simulink library "BEML_EMU_CBTCInterface_Lib"  (R2019b)
settings: Solver=VariableStepAuto  StartTime=0.0  StopTime=10.0  RelTol=1e-3
undefined symbols (not defined in the file): ATCCabActivation, ATCSBResetIndication, ATCZeroSpeed, ATOBrake, ATONotBrake, ATOStartIndication, ATOState, ATOTBDemand, ATOTraction, CabActive, DMI, Door1Inhibited, Door2Inhibited, Door3Inhibited, Door4Inhibited, Electrical, EmergencyDetrainmentDoorLocked, LeftDoorCloseATCReq, LeftDoorCloseIndicator, LeftDoorOpenATCReq, LeftHoldDoorClose, LeftSideDoorCloseRequest, LeftSideDoorEnable, LeftSideDoorOpenRequest, NeutralSection, NoEmergencyBrakeOrder, NoServiceBrake, NotImmobilise, OnBoard, Platform, PowerOn, RightDoorCloseATCReq, RightDoorCloseIndicator, RightDoorOpenATCReq, RightHoldDoorClose, RightSideDoorCloseRequest, RightSideDoorEnable, RightSideDoorOpenRequest, RollbackDetected, ROSIndication, TCMS, TractionForward, u2, u3, u4, UTOModeActive, UTOPBIndicator, WakeUpCommand
libraries: simulink x8, LatchesLib x4
settings Model: Creator=rleighton  LastModifiedBy=hinganes
settings DataIOCC: ReturnWorkspaceOutputs=off
settings DebuggingCC: ArithmeticOperatorsInVariantConditions=warning
settings SFSimCC: SimUseLocalCustomCode=off  CustomCodeUndefinedFunction=UseInterfaceOnly
settings RTWCC: RTWUseLocalCustomCode=off

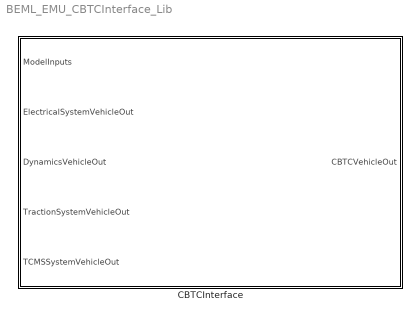
== system BEML_EMU_CBTCInterface_Lib ==
  CBTCInterface : Subsystem  SystemSampleTime=0.001

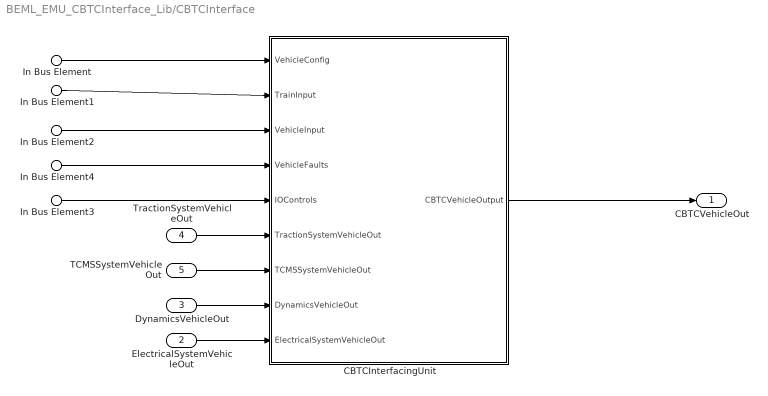
== system BEML_EMU_CBTCInterface_Lib/CBTCInterface ==
  In Bus Element : Inport  PortName=ModelInputs  Element=ProcessedVehicleConfig
  In Bus Element1 : Inport  PortName=ModelInputs  Element=ProcessedTrainInput
  In Bus Element2 : Inport  PortName=ModelInputs  Element=ProcessedVehicleInput
  In Bus Element4 : Inport  PortName=ModelInputs  Element=VehicleModelFaults
  In Bus Element3 : Inport  PortName=ModelInputs  Element=InputControlStates
  ElectricalSystemVehicleOut : Inport  Port=2
  DynamicsVehicleOut : Inport  Port=3
  TractionSystemVehicleOut : Inport  Port=4
  TCMSSystemVehicleOut : Inport  Port=5
  CBTCInterfacingUnit : Subsystem  TreatAsAtomicUnit=on  SystemSampleTime=0.01
  CBTCVehicleOut : Outport  VectorParamsAs1DForOutWhenUnconnected=off
  wires:
  In Bus Element3/1 -> CBTCInterfacingUnit/5(IOControls)
  CBTCInterfacingUnit/1(CBTCVehicleOutput) -> CBTCVehicleOut/1
  TractionSystemVehicleOut/1 -> CBTCInterfacingUnit/6(TractionSystemVehicleOut)
  TCMSSystemVehicleOut/1 -> CBTCInterfacingUnit/7(TCMSSystemVehicleOut)
  In Bus Element/1 -> CBTCInterfacingUnit/1(VehicleConfig)
  In Bus Element4/1 -> CBTCInterfacingUnit/4(VehicleFaults)
  In Bus Element2/1 -> CBTCInterfacingUnit/3(VehicleInput)
  In Bus Element1/1 -> CBTCInterfacingUnit/2(TrainInput)
  DynamicsVehicleOut/1 -> CBTCInterfacingUnit/8(DynamicsVehicleOut)
  ElectricalSystemVehicleOut/1 -> CBTCInterfacingUnit/9(ElectricalSystemVehicleOut)

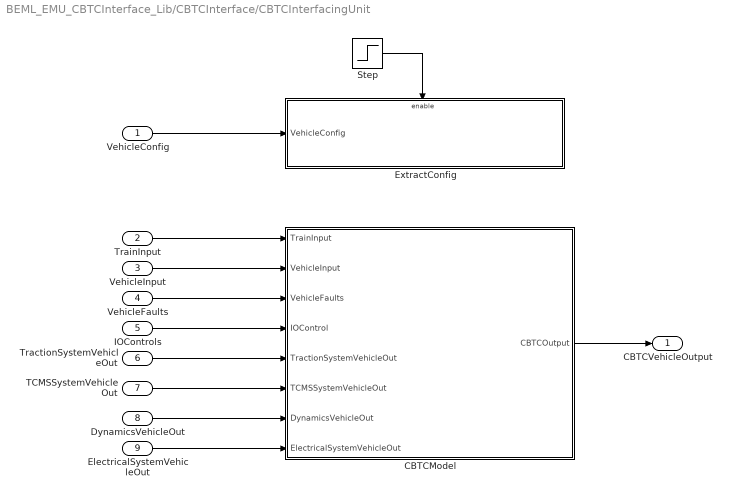
== system BEML_EMU_CBTCInterface_Lib/CBTCInterface/CBTCInterfacingUnit ==
  VehicleConfig : Inport  SampleTime=0.01
  TrainInput : Inport  Port=2  SampleTime=0.01
  VehicleInput : Inport  Port=3  SampleTime=0.01
  VehicleFaults : Inport  Port=4  SampleTime=0.01
  IOControls : Inport  Port=5
  TractionSystemVehicleOut : Inport  Port=6  SampleTime=0.01
  TCMSSystemVehicleOut : Inport  Port=7  SampleTime=0.01
  DynamicsVehicleOut : Inport  Port=8  SampleTime=0.01
  ElectricalSystemVehicleOut : Inport  Port=9  SampleTime=0.01
  CBTCModel : Subsystem
  ExtractConfig : Subsystem
  Step : Step  Before=1  After=0
  CBTCVehicleOutput : Outport  VectorParamsAs1DForOutWhenUnconnected=off
  wires:
  IOControls/1 -> CBTCModel/4(IOControl)
  TrainInput/1 -> CBTCModel/1(TrainInput)
  VehicleInput/1 -> CBTCModel/2(VehicleInput)
  TractionSystemVehicleOut/1 -> CBTCModel/5(TractionSystemVehicleOut)
  TCMSSystemVehicleOut/1 -> CBTCModel/6(TCMSSystemVehicleOut)
  VehicleConfig/1 -> ExtractConfig/1(VehicleConfig)
  Step/1 -> ExtractConfig/Enable
  VehicleFaults/1 -> CBTCModel/3(VehicleFaults)
  CBTCModel/1(CBTCOutput) -> CBTCVehicleOutput/1
  DynamicsVehicleOut/1 -> CBTCModel/7(DynamicsVehicleOut)
  ElectricalSystemVehicleOut/1 -> CBTCModel/8(ElectricalSystemVehicleOut)

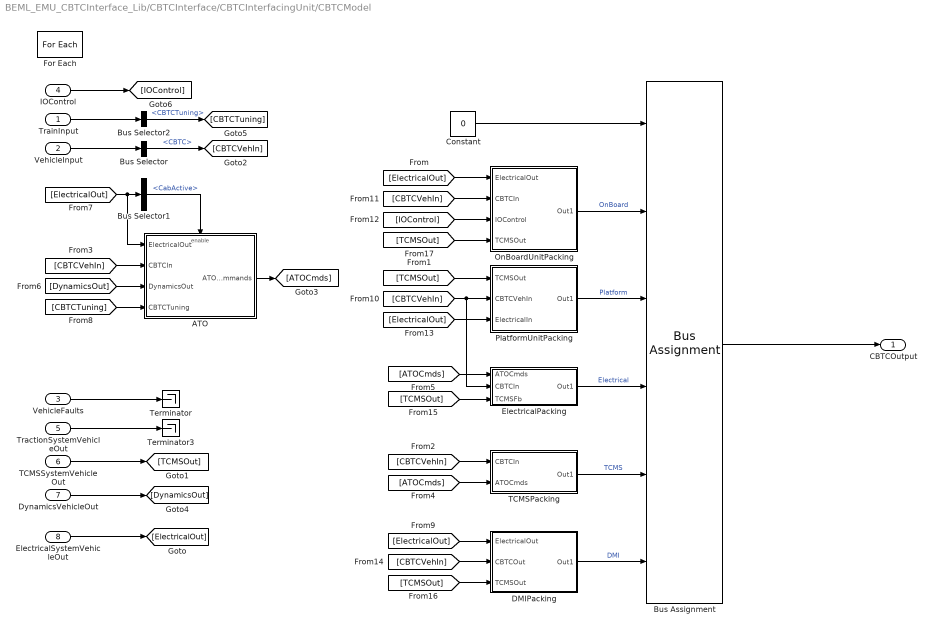
== system BEML_EMU_CBTCInterface_Lib/CBTCInterface/CBTCInterfacingUnit/CBTCModel ==
  TrainInput : Inport
  VehicleInput : Inport  Port=2  Partition=on  PartitionDimension=1  PartitionWidth=1  PartitionOffset=0
  VehicleFaults : Inport  Port=3  Partition=on  PartitionDimension=1  PartitionWidth=1  PartitionOffset=0
  IOControl : Inport  Port=4  Partition=on  PartitionDimension=1  PartitionWidth=1  PartitionOffset=0
  TractionSystemVehicleOut : Inport  Port=5  Partition=on  PartitionDimension=1  PartitionWidth=1  PartitionOffset=0
  TCMSSystemVehicleOut : Inport  Port=6  Partition=on  PartitionDimension=1  PartitionWidth=1  PartitionOffset=0
  DynamicsVehicleOut : Inport  Port=7  Partition=on  PartitionDimension=1  PartitionWidth=1  PartitionOffset=0
  ElectricalSystemVehicleOut : Inport  Port=8  Partition=on  PartitionDimension=1  PartitionWidth=1  PartitionOffset=0
  ATO : Subsystem
  Bus Assignment : BusAssignment  AssignedSignals=OnBoard,Platform,Electrical,TCMS,DMI
  Bus Selector : BusSelector  OutputSignals=CBTC
  Bus Selector1 : BusSelector  OutputSignals=TCMS.CabActive
  Bus Selector2 : BusSelector  OutputSignals=CBTCTuning
  Constant : Constant  Value=0  OutDataTypeStr=Bus: BD_CBTC_Out_Vehicle
  DMIPacking : Subsystem
  ElectricalPacking : Subsystem
  For Each : ForEach  DisableCoverage=on
  OnBoardUnitPacking : Subsystem
  PlatformUnitPacking : Subsystem
  TCMSPacking : Subsystem
  Terminator : Terminator
  Terminator3 : Terminator
  CBTCOutput : Outport  ConcatenationDimension=1  VectorParamsAs1DForOutWhenUnconnected=off
  wires:
  [TCMSOut] -> OnBoardUnitPacking/4(TCMSOut)
  [TCMSOut] -> DMIPacking/3(TCMSOut)
  [TCMSOut] -> ElectricalPacking/3(TCMSFb)
  [CBTCVehIn] -> DMIPacking/2(CBTCOut)
  [ElectricalOut] -> PlatformUnitPacking/3(ElectricalIn)
  [IOControl] -> OnBoardUnitPacking/3(IOControl)
  IOControl/1 -> [IOControl]
  [CBTCVehIn] -> OnBoardUnitPacking/2(CBTCIn)
  [CBTCVehIn] -> PlatformUnitPacking/2(CBTCVehIn), ElectricalPacking/2(CBTCIn)
  ElectricalSystemVehicleOut/1 -> [ElectricalOut]
  Bus Assignment/1 -> CBTCOutput/1
  Bus Selector/1 -> [CBTCVehIn]  "<CBTC>"
  TrainInput/1 -> Bus Selector2/1
  VehicleInput/1 -> Bus Selector/1
  VehicleFaults/1 -> Terminator/1
  TractionSystemVehicleOut/1 -> Terminator3/1
  TCMSSystemVehicleOut/1 -> [TCMSOut]
  DynamicsVehicleOut/1 -> [DynamicsOut]
  OnBoardUnitPacking/1(Out1) -> Bus Assignment/2  "OnBoard"
  [ElectricalOut] -> OnBoardUnitPacking/1(ElectricalOut)
  Constant/1 -> Bus Assignment/1
  PlatformUnitPacking/1(Out1) -> Bus Assignment/3  "Platform"
  [TCMSOut] -> PlatformUnitPacking/1(TCMSOut)
  ElectricalPacking/1(Out1) -> Bus Assignment/4  "Electrical"
  TCMSPacking/1(Out1) -> Bus Assignment/5  "TCMS"
  [CBTCVehIn] -> TCMSPacking/1(CBTCIn)
  [CBTCVehIn] -> ATO/2(CBTCIn)
  ATO/1(ATOCommands) -> [ATOCmds]
  [ATOCmds] -> TCMSPacking/2(ATOCmds)
  [ATOCmds] -> ElectricalPacking/1(ATOCmds)
  [DynamicsOut] -> ATO/3(DynamicsOut)
  [ElectricalOut] -> ATO/1(ElectricalOut), Bus Selector1/1
  Bus Selector1/1 -> ATO/Enable  "<CabActive>"
  Bus Selector2/1 -> [CBTCTuning]  "<CBTCTuning>"
  [CBTCTuning] -> ATO/4(CBTCTuning)
  DMIPacking/1(Out1) -> Bus Assignment/6  "DMI"
  [ElectricalOut] -> DMIPacking/1(ElectricalOut)

== system BEML_EMU_CBTCInterface_Lib/CBTCInterface/CBTCInterfacingUnit/ExtractConfig ==
  VehicleConfig : Inport
  Enable : EnablePort
  ExtractConfig : Subsystem
  wires:
  VehicleConfig/1 -> ExtractConfig/1(VehicleConfig)

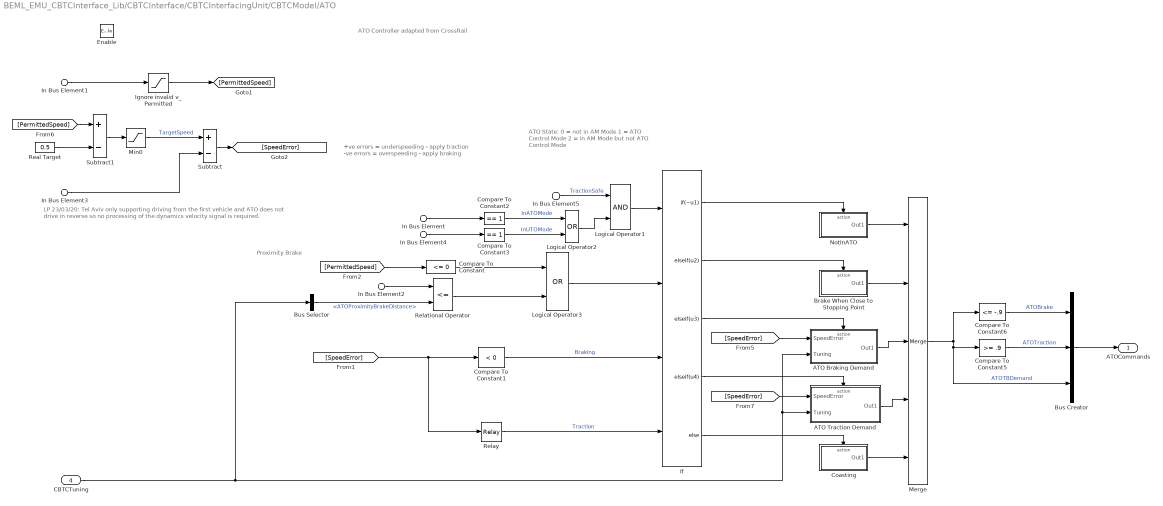
== system BEML_EMU_CBTCInterface_Lib/CBTCInterface/CBTCInterfacingUnit/CBTCModel/ATO ==
  note: ATO Controller adapted from CrossRail
  note: ATO State:
      | 0 = not in AM Mode
      | 1 = ATO Control Mode
      | 2 = in AM Mode but not ATO Control Mode
  note: +ve errors = underspeeding - apply traction
      | -ve errors = overspeeding - apply braking
  note: LP 23/03/20: Tel Aviv only supporting driving from the first vehicle and ATO does
      | not drive in reverse so no processing of the dynamics velocity signal is required.
  note: Proximity Brake
  In Bus Element5 : Inport  PortName=ElectricalOut  Element=Traction.TractionSafe
  In Bus Element : Inport  Port=2  PortName=CBTCIn  Element=OnBoard.ATOState
  In Bus Element1 : Inport  Port=2  PortName=CBTCIn  Element=OnBoard.ATOPermittedSpeed
  In Bus Element2 : Inport  Port=2  PortName=CBTCIn  Element=OnBoard.ATOPermittedDistance
  In Bus Element4 : Inport  Port=2  PortName=CBTCIn  Element=OnBoard.UTOModeActive
  In Bus Element3 : Inport  Port=3  PortName=DynamicsOut  Element=Inertia.Velocity
  CBTCTuning : Inport  Port=4
  Enable : EnablePort  StatesWhenEnabling=reset
  ATO Braking Demand : Subsystem  TreatAsAtomicUnit=on
  ATO Traction Demand : Subsystem  TreatAsAtomicUnit=on
  Brake When Close to Stopping Point : Subsystem  TreatAsAtomicUnit=on
  Bus Creator : BusCreator  Inputs=3
  Bus Selector : BusSelector  OutputSignals=ATOProximityBrakeDistance
  Coasting : Subsystem  TreatAsAtomicUnit=on
  Compare To Constant : simulink/Logic and Bit Operations/Compare To Constant  relop=<=  const=0  OutDataTypeStr=boolean
  Compare To Constant1 : simulink/Logic and Bit Operations/Compare To Constant  relop=<  const=0  OutDataTypeStr=boolean
  Compare To Constant2 : simulink/Logic and Bit Operations/Compare To Constant  relop===  const=1  OutDataTypeStr=boolean
  Compare To Constant3 : simulink/Logic and Bit Operations/Compare To Constant  relop===  const=1  OutDataTypeStr=boolean
  Compare To Constant5 : simulink/Logic and Bit Operations/Compare To Constant  relop=>=  const=.9  OutDataTypeStr=boolean
  Compare To Constant6 : simulink/Logic and Bit Operations/Compare To Constant  relop=<=  const=-.9  OutDataTypeStr=boolean
  If : If  NumInputs=4  IfExpression=~u1  ElseIfExpressions=u2,u3,u4
  Ignore invalid v_Permitted : Saturate  UpperLimit=80/3.6  LowerLimit=0
  Logical Operator1 : Logic  AllPortsSameDT=off  OutDataTypeStr=boolean
  Logical Operator2 : Logic  Operator=OR  AllPortsSameDT=off  OutDataTypeStr=boolean
  Logical Operator3 : Logic  Operator=OR  AllPortsSameDT=off  OutDataTypeStr=boolean
  Merge : Merge  Inputs=5
  Min0 : Saturate  UpperLimit=inf  LowerLimit=0
  NotInATO : Subsystem  TreatAsAtomicUnit=on
  Real Target : Constant  Value=0.5
  Relational Operator : RelationalOperator  Operator=<=  OutDataTypeStr=boolean  RndMeth=Simplest
  Relay : Relay  OnSwitchValue=0.5  OffSwitchValue=0.05  OutDataTypeStr=boolean
  Subtract : Sum  Inputs=+-
  Subtract1 : Sum  Inputs=+-
  ATOCommands : Outport
  wires:
  In Bus Element4/1 -> Compare To Constant3/1
  Compare To Constant3/1 -> Logical Operator2/2  "InUTOMode"
  Logical Operator2/1 -> Logical Operator1/2
  Compare To Constant2/1 -> Logical Operator2/1  "InATOMode"
  Merge/1 -> Bus Creator/3, Compare To Constant5/1, Compare To Constant6/1  "ATOTBDemand"
  Bus Creator/1 -> ATOCommands/1
  Relational Operator/1 -> Logical Operator3/2
  ATO Braking Demand/1(Out1) -> Merge/3
  Compare To Constant5/1 -> Bus Creator/2  "ATOTraction"
  Compare To Constant6/1 -> Bus Creator/1  "ATOBrake"
  [SpeedError] -> Relay/1, Compare To Constant1/1
  CBTCTuning/1 -> ATO Braking Demand/2(Tuning), ATO Traction Demand/2(Tuning), Bus Selector/1
  Compare To Constant1/1 -> If/3  "Braking"
  If/3 -> ATO Braking Demand/Action
  Ignore invalid v_Permitted/1 -> [PermittedSpeed]
  Subtract/1 -> [SpeedError]
  Relay/1 -> If/4  "Traction"
  [SpeedError] -> ATO Braking Demand/1(SpeedError)
  In Bus Element2/1 -> Relational Operator/1
  Compare To Constant/1 -> Logical Operator3/1
  If/4 -> ATO Traction Demand/Action
  Logical Operator3/1 -> If/2
  [SpeedError] -> ATO Traction Demand/1(SpeedError)
  In Bus Element3/1 -> Subtract/2
  In Bus Element1/1 -> Ignore invalid v_Permitted/1
  If/5 -> Coasting/Action
  ATO Traction Demand/1(Out1) -> Merge/4
  If/2 -> Brake When Close to Stopping Point/Action
  Real Target/1 -> Subtract1/2
  Brake When Close to Stopping Point/1(Out1) -> Merge/2
  Coasting/1(Out1) -> Merge/5
  [PermittedSpeed] -> Compare To Constant/1
  [PermittedSpeed] -> Subtract1/1
  If/1 -> NotInATO/Action
  NotInATO/1(Out1) -> Merge/1
  Logical Operator1/1 -> If/1
  Min0/1 -> Subtract/1  "TargetSpeed"
  In Bus Element5/1 -> Logical Operator1/1  "TractionSafe"
  In Bus Element/1 -> Compare To Constant2/1
  Subtract1/1 -> Min0/1
  Bus Selector/1 -> Relational Operator/2  "<ATOProximityBrakeDistance>"

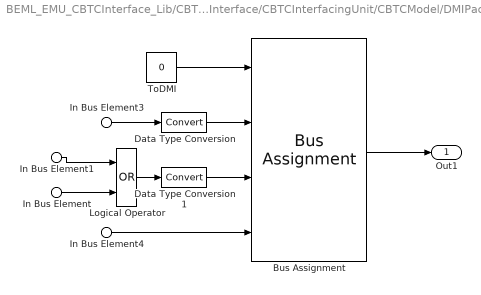
== system BEML_EMU_CBTCInterface_Lib/CBTCInterface/CBTCInterfacingUnit/CBTCModel/DMIPacking ==
  In Bus Element1 : Inport  PortName=ElectricalOut  Element=SignalSys.CabActive
  In Bus Element3 : Inport  PortName=ElectricalOut  Element=SignalSys.DMIPower
  In Bus Element : Inport  Port=2  PortName=CBTCOut  Element=OnBoard.ATCCabActivation
  In Bus Element4 : Inport  Port=3  PortName=TCMSOut  Element=Control.ElectricalSystem.TrainInNeutralSection
  Bus Assignment : BusAssignment  AssignedSignals=PowerOn,CabActive,NeutralSection
  Data Type Conversion : DataTypeConversion
  Data Type Conversion1 : DataTypeConversion
  Logical Operator : Logic  Operator=OR  AllPortsSameDT=off  OutDataTypeStr=boolean
  ToDMI : Constant  Value=0  OutDataTypeStr=Bus: BD_CBTC_Out_Vehicle_DMI
  Out1 : Outport
  wires:
  In Bus Element4/1 -> Bus Assignment/4
  In Bus Element/1 -> Logical Operator/2
  Logical Operator/1 -> Data Type Conversion1/1
  Data Type Conversion1/1 -> Bus Assignment/3
  Data Type Conversion/1 -> Bus Assignment/2
  Bus Assignment/1 -> Out1/1
  ToDMI/1 -> Bus Assignment/1
  In Bus Element1/1 -> Logical Operator/1
  In Bus Element3/1 -> Data Type Conversion/1

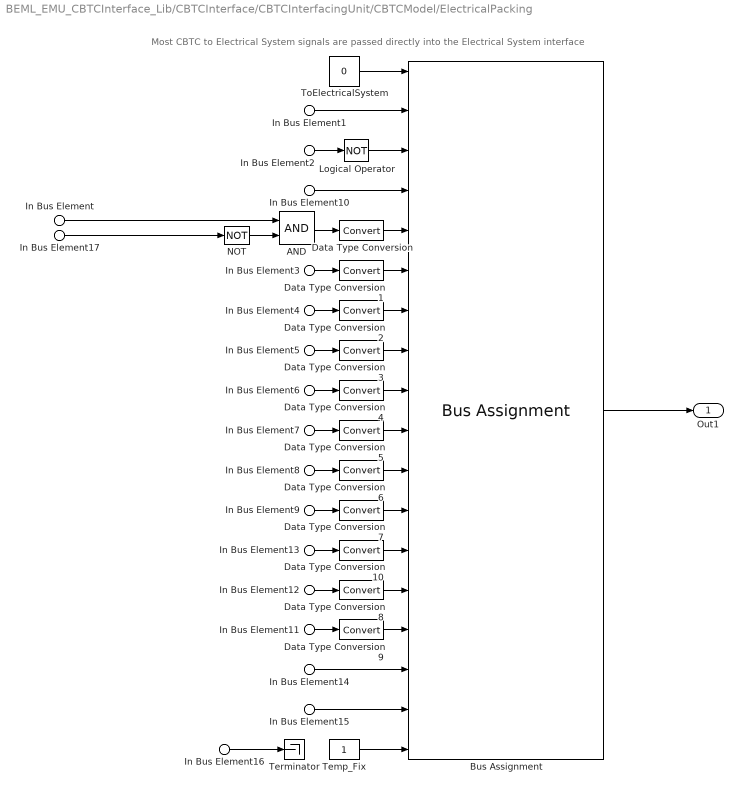
== system BEML_EMU_CBTCInterface_Lib/CBTCInterface/CBTCInterfacingUnit/CBTCModel/ElectricalPacking ==
  note: Most CBTC to Electrical System signals are passed directly into the Electrical System interface
  In Bus Element1 : Inport  PortName=ATOCmds  Element=ATOTraction
  In Bus Element2 : Inport  PortName=ATOCmds  Element=ATOBrake
  In Bus Element10 : Inport  PortName=ATOCmds  Element=ATOTBDemand
  In Bus Element : Inport  Port=2  PortName=CBTCIn  Element=OnBoard.NoEmergencyBrakeOrder
  In Bus Element3 : Inport  Port=2  PortName=CBTCIn  Element=OnBoard.ROSIndicator
  In Bus Element4 : Inport  Port=2  PortName=CBTCIn  Element=OnBoard.ATCSBResetIndicator
  In Bus Element5 : Inport  Port=2  PortName=CBTCIn  Element=OnBoard.ATOStartIndicator
  In Bus Element6 : Inport  Port=2  PortName=CBTCIn  Element=OnBoard.LeftHoldDoorClose
  In Bus Element7 : Inport  Port=2  PortName=CBTCIn  Element=OnBoard.RightHoldDoorClose
  In Bus Element8 : Inport  Port=2  PortName=CBTCIn  Element=OnBoard.ZeroSpeed
  In Bus Element9 : Inport  Port=2  PortName=CBTCIn  Element=OnBoard.WakeUpCommand
  In Bus Element11 : Inport  Port=2  PortName=CBTCIn  Element=OnBoard.ATCCabActivation
  In Bus Element12 : Inport  Port=2  PortName=CBTCIn  Element=OnBoard.UTOPBIndicator
  In Bus Element13 : Inport  Port=2  PortName=CBTCIn  Element=OnBoard.UTOModeActive
  In Bus Element14 : Inport  Port=2  PortName=CBTCIn  Element=OnBoard.ImmobilisationState
  In Bus Element15 : Inport  Port=2  PortName=CBTCIn  Element=OnBoard.TractionForward
  In Bus Element16 : Inport  Port=2  PortName=CBTCIn  Element=OnBoard.EmergencyDetrainmentDoorLocked
  In Bus Element17 : Inport  Port=3  PortName=TCMSFb  Element=Display.DoorSystem.UnexpectedDoorOpeningDetectedByCC
  AND : Logic  AllPortsSameDT=off  OutDataTypeStr=boolean
  Bus Assignment : BusAssignment  AssignedSignals=ATOTraction,ATONotBrake,ATOTBDemand,NoEmergencyBrakeOrder,ROSIndication,ATCSBResetIndication,ATOStartIndication,LeftHoldDoorClose,RightHoldDoorClose,ATCZeroSpeed,WakeUpCommand,UTOModeActive,UTOPBIndicator,ATCCabActivation,NotImmobilise,TractionForward,EmergencyDetrainmentDoorLocked
  Data Type Conversion{,1..10} (11 alike) : DataTypeConversion
  Logical Operator : Logic  Operator=NOT  AllPortsSameDT=off  OutDataTypeStr=boolean
  NOT : Logic  Operator=NOT  AllPortsSameDT=off  OutDataTypeStr=boolean
  Temp_Fix : Constant
  Terminator : Terminator
  ToElectricalSystem : Constant  Value=0  OutDataTypeStr=Bus: BD_CBTC_Out_Vehicle_Electrical
  Out1 : Outport
  wires:
  In Bus Element17/1 -> NOT/1
  In Bus Element/1 -> AND/1
  NOT/1 -> AND/2
  Temp_Fix/1 -> Bus Assignment/18
  In Bus Element16/1 -> Terminator/1
  In Bus Element15/1 -> Bus Assignment/17
  In Bus Element14/1 -> Bus Assignment/16
  Data Type Conversion9/1 -> Bus Assignment/15
  Data Type Conversion8/1 -> Bus Assignment/14
  Data Type Conversion10/1 -> Bus Assignment/13
  Data Type Conversion7/1 -> Bus Assignment/12
  Data Type Conversion6/1 -> Bus Assignment/11
  Data Type Conversion5/1 -> Bus Assignment/10
  Data Type Conversion4/1 -> Bus Assignment/9
  Data Type Conversion3/1 -> Bus Assignment/8
  Data Type Conversion2/1 -> Bus Assignment/7
  Data Type Conversion1/1 -> Bus Assignment/6
  Data Type Conversion/1 -> Bus Assignment/5
  In Bus Element10/1 -> Bus Assignment/4
  In Bus Element13/1 -> Data Type Conversion10/1
  In Bus Element11/1 -> Data Type Conversion9/1
  In Bus Element12/1 -> Data Type Conversion8/1
  In Bus Element9/1 -> Data Type Conversion7/1
  In Bus Element8/1 -> Data Type Conversion6/1
  In Bus Element7/1 -> Data Type Conversion5/1
  In Bus Element6/1 -> Data Type Conversion4/1
  In Bus Element5/1 -> Data Type Conversion3/1
  In Bus Element4/1 -> Data Type Conversion2/1
  In Bus Element3/1 -> Data Type Conversion1/1
  AND/1 -> Data Type Conversion/1
  ToElectricalSystem/1 -> Bus Assignment/1
  Bus Assignment/1 -> Out1/1
  In Bus Element1/1 -> Bus Assignment/2
  In Bus Element2/1 -> Logical Operator/1
  Logical Operator/1 -> Bus Assignment/3

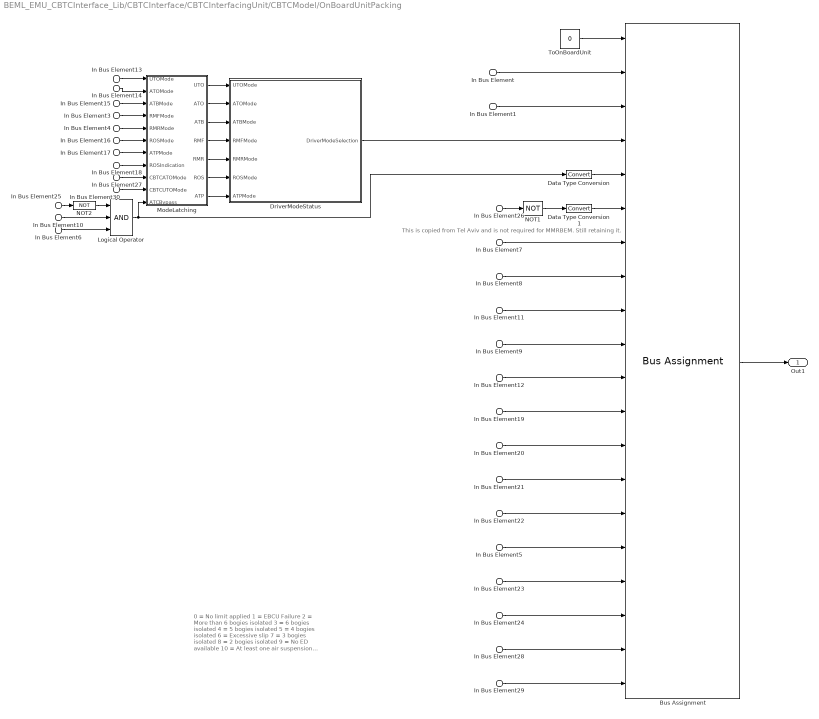
== system BEML_EMU_CBTCInterface_Lib/CBTCInterface/CBTCInterfacingUnit/CBTCModel/OnBoardUnitPacking ==
  note: This is copied from Tel Aviv and is not required for MMRBEM. Still retaining it.
  note: 0 = No limit applied
      | 1 = EBCU Failure
      | 2 = More than 6 bogies isolated
      | 3 = 6 bogies isolated
      | 4 = 5 bogies isolated
      | 5 = 4 bogies isolated
      | 6 = Excessive slip
      | 7 = 3 bogies isolated
      | 8 = 2 bogies isolated
      | 9 = No ED available
      | 10 = At least one air suspension deflated
  In Bus Element : Inport  PortName=ElectricalOut  Element=SignalSys.ATCPower
  In Bus Element6 : Inport  PortName=ElectricalOut  Element=SignalSys.ATCPower
  In Bus Element1 : Inport  PortName=ElectricalOut  Element=SignalSys.CabActive
  In Bus Element3 : Inport  PortName=ElectricalOut  Element=SignalSys.RMFMode
  In Bus Element4 : Inport  PortName=ElectricalOut  Element=SignalSys.RMRMode
  In Bus Element7 : Inport  PortName=ElectricalOut  Element=SignalSys.ATOStartPB
  In Bus Element8 : Inport  PortName=ElectricalOut  Element=SignalSys.ATCSafetyBrakeResetPB
  In Bus Element11 : Inport  PortName=ElectricalOut  Element=SignalSys.NotSafetyBrake
  In Bus Element13 : Inport  PortName=ElectricalOut  Element=SignalSys.UTOMode
  In Bus Element14 : Inport  PortName=ElectricalOut  Element=SignalSys.ATOMode
  In Bus Element15 : Inport  PortName=ElectricalOut  Element=SignalSys.ATBMode
  In Bus Element16 : Inport  PortName=ElectricalOut  Element=SignalSys.ROSMode
  In Bus Element17 : Inport  PortName=ElectricalOut  Element=SignalSys.ATPMode
  In Bus Element20 : Inport  PortName=ElectricalOut  Element=SignalSys.EmergencyDoorNotOpen
  In Bus Element21 : Inport  PortName=ElectricalOut  Element=SignalSys.WakeUpStatus
  In Bus Element12 : Inport  PortName=ElectricalOut  Element=SignalSys.TrainDoorClosedAndLocked
  In Bus Element22 : Inport  PortName=ElectricalOut  Element=SignalSys.UTOStartPB
  In Bus Element9 : Inport  PortName=ElectricalOut  Element=SignalSys.DoorEnableBypass
  In Bus Element5 : Inport  PortName=ElectricalOut  Element=SignalSys.PassengerEmergencyAlarm
  In Bus Element23 : Inport  PortName=ElectricalOut  Element=SignalSys.FireSmokeInd
  In Bus Element24 : Inport  PortName=ElectricalOut  Element=SignalSys.MechanicalCoupling
  In Bus Element25 : Inport  PortName=ElectricalOut  Element=SignalSys.NoATCBypass
  In Bus Element26 : Inport  PortName=ElectricalOut  Element=SignalSys.TBCInFSB
  In Bus Element10 : Inport  PortName=ElectricalOut  Element=TCMS.CabActive
  In Bus Element18 : Inport  Port=2  PortName=CBTCIn  Element=OnBoard.ROSIndicator
  In Bus Element27 : Inport  Port=2  PortName=CBTCIn  Element=OnBoard.ATOState
  In Bus Element30 : Inport  Port=2  PortName=CBTCIn  Element=OnBoard.UTOModeActive
  In Bus Element19 : Inport  Port=3  PortName=IOControl  Element=ModeSelector
  In Bus Element28 : Inport  Port=4  PortName=TCMSOut  Element=Control.TractionSBraking.TCMSSpeedLimit
  In Bus Element29 : Inport  Port=4  PortName=TCMSOut  Element=Control.TractionSBraking.TCMSSpeedLimitCause
  Bus Assignment : BusAssignment  AssignedSignals=PowerSupply,CabinActivation,DriverModeSelection,ATCBypassState,TBCPosition,ATOStartButton,ATCSBResetButton,NoEmergencyBrake,NoDoorEnableBypass,TrainDoorClosedAndLocked,ModeSelectorPosition,EmergencyDoorNotOpen,WakeUpStatus,UTOStartButton,PassengerEmergencyAlarm,FireSmokeInd,MechanicalCoupling,TCMSSpeedLimit,TCMSSpeedLimitCause
  Data Type Conversion : DataTypeConversion
  Data Type Conversion1 : DataTypeConversion
  DriverModeStatus : Subsystem
  Logical Operator : Logic  Inputs=3  AllPortsSameDT=off  OutDataTypeStr=boolean
  ModeLatching : Subsystem
  NOT1 : Logic  Operator=NOT  AllPortsSameDT=off  OutDataTypeStr=boolean
  NOT2 : Logic  Operator=NOT  AllPortsSameDT=off  OutDataTypeStr=boolean
  ToOnBoardUnit : Constant  Value=0  OutDataTypeStr=Bus: BD_CBTC_Out_Vehicle_Onboard
  Out1 : Outport
  wires:
  In Bus Element30/1 -> ModeLatching/10(CBTCUTOMode)
  In Bus Element29/1 -> Bus Assignment/20
  In Bus Element28/1 -> Bus Assignment/19
  In Bus Element6/1 -> Logical Operator/3
  In Bus Element10/1 -> Logical Operator/2
  NOT2/1 -> Logical Operator/1
  Logical Operator/1 -> Data Type Conversion/1, ModeLatching/11(ATCBypass)
  In Bus Element24/1 -> Bus Assignment/18
  In Bus Element23/1 -> Bus Assignment/17
  In Bus Element5/1 -> Bus Assignment/16
  In Bus Element22/1 -> Bus Assignment/15
  In Bus Element21/1 -> Bus Assignment/14
  In Bus Element20/1 -> Bus Assignment/13
  In Bus Element27/1 -> ModeLatching/9(CBTCATOMode)
  In Bus Element19/1 -> Bus Assignment/12
  In Bus Element18/1 -> ModeLatching/8(ROSIndication)
  ModeLatching/7(ATP) -> DriverModeStatus/7(ATPMode)
  ModeLatching/6(ROS) -> DriverModeStatus/6(ROSMode)
  ModeLatching/5(RMR) -> DriverModeStatus/5(RMRMode)
  ModeLatching/4(RMF) -> DriverModeStatus/4(RMFMode)
  ModeLatching/3(ATB) -> DriverModeStatus/3(ATBMode)
  ModeLatching/2(ATO) -> DriverModeStatus/2(ATOMode)
  ModeLatching/1(UTO) -> DriverModeStatus/1(UTOMode)
  In Bus Element17/1 -> ModeLatching/7(ATPMode)
  In Bus Element16/1 -> ModeLatching/6(ROSMode)
  In Bus Element15/1 -> ModeLatching/3(ATBMode)
  In Bus Element14/1 -> ModeLatching/2(ATOMode)
  Bus Assignment/1 -> Out1/1
  ToOnBoardUnit/1 -> Bus Assignment/1
  In Bus Element/1 -> Bus Assignment/2
  In Bus Element1/1 -> Bus Assignment/3
  DriverModeStatus/1(DriverModeSelection) -> Bus Assignment/4
  In Bus Element13/1 -> ModeLatching/1(UTOMode)
  In Bus Element3/1 -> ModeLatching/4(RMFMode)
  In Bus Element4/1 -> ModeLatching/5(RMRMode)
  In Bus Element25/1 -> NOT2/1
  In Bus Element26/1 -> NOT1/1
  NOT1/1 -> Data Type Conversion1/1
  In Bus Element7/1 -> Bus Assignment/7
  In Bus Element8/1 -> Bus Assignment/8
  In Bus Element9/1 -> Bus Assignment/10
  In Bus Element11/1 -> Bus Assignment/9
  In Bus Element12/1 -> Bus Assignment/11
  Data Type Conversion/1 -> Bus Assignment/5
  Data Type Conversion1/1 -> Bus Assignment/6

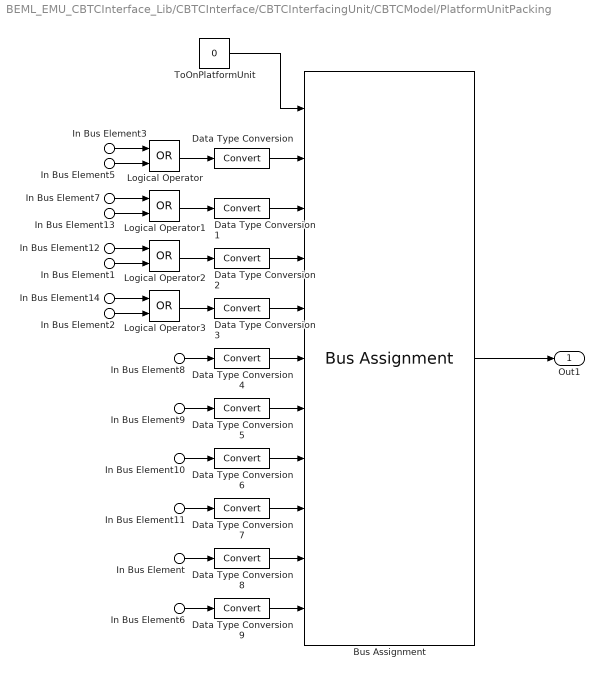
== system BEML_EMU_CBTCInterface_Lib/CBTCInterface/CBTCInterfacingUnit/CBTCModel/PlatformUnitPacking ==
  In Bus Element8 : Inport  PortName=TCMSOut  Element=Control.DoorSystem.DoorRight1Isolation
  In Bus Element9 : Inport  PortName=TCMSOut  Element=Control.DoorSystem.DoorLeft1Isolation
  In Bus Element10 : Inport  PortName=TCMSOut  Element=Control.DoorSystem.DoorRight2Isolation
  In Bus Element11 : Inport  PortName=TCMSOut  Element=Control.DoorSystem.DoorLeft2Isolation
  In Bus Element : Inport  Port=2  PortName=CBTCVehIn  Element=Platform.LeftSideDoorEnable
  In Bus Element6 : Inport  Port=2  PortName=CBTCVehIn  Element=Platform.RightSideDoorEnable
  In Bus Element5 : Inport  Port=2  PortName=CBTCVehIn  Element=Platform.OpenLeftTrainDoors
  In Bus Element13 : Inport  Port=2  PortName=CBTCVehIn  Element=Platform.OpenRightTrainDoors
  In Bus Element1 : Inport  Port=2  PortName=CBTCVehIn  Element=Platform.CloseLeftTrainDoors
  In Bus Element2 : Inport  Port=2  PortName=CBTCVehIn  Element=Platform.CloseRightTrainDoors
  In Bus Element7 : Inport  Port=3  PortName=ElectricalIn  Element=SignalSys.RightDoorOpenPB
  In Bus Element12 : Inport  Port=3  PortName=ElectricalIn  Element=SignalSys.LeftDoorClosePB
  In Bus Element14 : Inport  Port=3  PortName=ElectricalIn  Element=SignalSys.RightDoorClosePB
  In Bus Element3 : Inport  Port=3  PortName=ElectricalIn  Element=SignalSys.LeftDoorOpenPB
  Bus Assignment : BusAssignment  AssignedSignals=LeftSideDoorOpenRequest,RightSideDoorOpenRequest,LeftSideDoorCloseRequest,RightSideDoorCloseRequest,Door1Inhibited,Door2Inhibited,Door3Inhibited,Door4Inhibited,LeftSideDoorEnable,RightSideDoorEnable
  Data Type Conversion{,1..9} (10 alike) : DataTypeConversion
  Logical Operator{,1..3} (4 alike) : Logic  Operator=OR  AllPortsSameDT=off  OutDataTypeStr=boolean
  ToOnPlatformUnit : Constant  Value=0  OutDataTypeStr=Bus: BD_CBTC_Out_Vehicle_Platform
  Out1 : Outport
  wires:
  In Bus Element14/1 -> Logical Operator3/1
  In Bus Element12/1 -> Logical Operator2/1
  In Bus Element3/1 -> Logical Operator/1
  In Bus Element7/1 -> Logical Operator1/1
  Logical Operator3/1 -> Data Type Conversion3/1
  Logical Operator2/1 -> Data Type Conversion2/1
  Logical Operator1/1 -> Data Type Conversion1/1
  Logical Operator/1 -> Data Type Conversion/1
  Data Type Conversion2/1 -> Bus Assignment/4
  Data Type Conversion3/1 -> Bus Assignment/5
  In Bus Element1/1 -> Logical Operator2/2
  In Bus Element2/1 -> Logical Operator3/2
  In Bus Element13/1 -> Logical Operator1/2
  In Bus Element5/1 -> Logical Operator/2
  Data Type Conversion9/1 -> Bus Assignment/11
  Data Type Conversion8/1 -> Bus Assignment/10
  In Bus Element6/1 -> Data Type Conversion9/1
  In Bus Element/1 -> Data Type Conversion8/1
  Data Type Conversion7/1 -> Bus Assignment/9
  Data Type Conversion6/1 -> Bus Assignment/8
  Data Type Conversion5/1 -> Bus Assignment/7
  Data Type Conversion4/1 -> Bus Assignment/6
  Data Type Conversion1/1 -> Bus Assignment/3
  Data Type Conversion/1 -> Bus Assignment/2
  ToOnPlatformUnit/1 -> Bus Assignment/1
  Bus Assignment/1 -> Out1/1
  In Bus Element8/1 -> Data Type Conversion4/1
  In Bus Element9/1 -> Data Type Conversion5/1
  In Bus Element10/1 -> Data Type Conversion6/1
  In Bus Element11/1 -> Data Type Conversion7/1

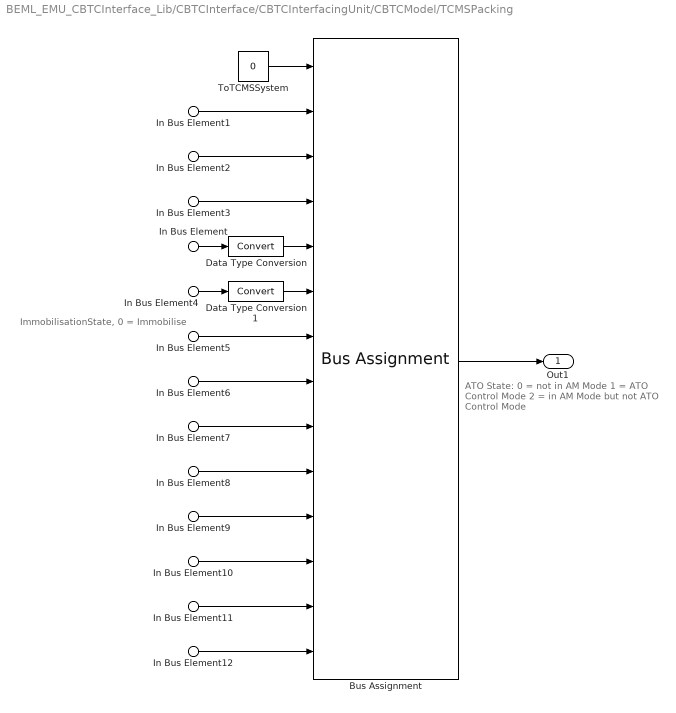
== system BEML_EMU_CBTCInterface_Lib/CBTCInterface/CBTCInterfacingUnit/CBTCModel/TCMSPacking ==
  note: ImmobilisationState, 0 = Immobilise
  note: ATO State:
      | 0 = not in AM Mode
      | 1 = ATO Control Mode
      | 2 = in AM Mode but not ATO Control Mode
  In Bus Element : Inport  PortName=CBTCIn  Element=OnBoard.NoServiceBrakeOrder
  In Bus Element5 : Inport  PortName=CBTCIn  Element=OnBoard.ATOState
  In Bus Element4 : Inport  PortName=CBTCIn  Element=OnBoard.ImmobilisationState
  In Bus Element6 : Inport  PortName=CBTCIn  Element=OnBoard.RollbackDetected
  In Bus Element7 : Inport  PortName=CBTCIn  Element=Platform.LeftDoorCloseIndicator
  In Bus Element8 : Inport  PortName=CBTCIn  Element=Platform.RightDoorCloseIndicator
  In Bus Element9 : Inport  PortName=CBTCIn  Element=Platform.OpenLeftTrainDoors
  In Bus Element10 : Inport  PortName=CBTCIn  Element=Platform.OpenRightTrainDoors
  In Bus Element11 : Inport  PortName=CBTCIn  Element=Platform.CloseLeftTrainDoors
  In Bus Element12 : Inport  PortName=CBTCIn  Element=Platform.CloseRightTrainDoors
  In Bus Element1 : Inport  Port=2  PortName=ATOCmds  Element=ATOTraction
  In Bus Element2 : Inport  Port=2  PortName=ATOCmds  Element=ATOBrake
  In Bus Element3 : Inport  Port=2  PortName=ATOCmds  Element=ATOTBDemand
  Bus Assignment : BusAssignment  AssignedSignals=ATOTraction,ATOBrake,ATOTBDemand,NoServiceBrake,NotImmobilise,ATOState,RollbackDetected,LeftDoorCloseIndicator,RightDoorCloseIndicator,LeftDoorOpenATCReq,RightDoorOpenATCReq,LeftDoorCloseATCReq,RightDoorCloseATCReq
  Data Type Conversion : DataTypeConversion
  Data Type Conversion1 : DataTypeConversion
  ToTCMSSystem : Constant  Value=0  OutDataTypeStr=Bus: BD_CBTC_Out_Vehicle_TCMS
  Out1 : Outport
  wires:
  In Bus Element12/1 -> Bus Assignment/14
  In Bus Element11/1 -> Bus Assignment/13
  In Bus Element10/1 -> Bus Assignment/12
  In Bus Element9/1 -> Bus Assignment/11
  In Bus Element7/1 -> Bus Assignment/9
  In Bus Element8/1 -> Bus Assignment/10
  In Bus Element6/1 -> Bus Assignment/8
  In Bus Element2/1 -> Bus Assignment/3
  In Bus Element1/1 -> Bus Assignment/2
  Bus Assignment/1 -> Out1/1
  ToTCMSSystem/1 -> Bus Assignment/1
  In Bus Element3/1 -> Bus Assignment/4
  In Bus Element/1 -> Data Type Conversion/1
  Data Type Conversion/1 -> Bus Assignment/5
  In Bus Element4/1 -> Data Type Conversion1/1
  Data Type Conversion1/1 -> Bus Assignment/6
  In Bus Element5/1 -> Bus Assignment/7

== system BEML_EMU_CBTCInterface_Lib/CBTCInterface/CBTCInterfacingUnit/ExtractConfig/ExtractConfig ==
  VehicleConfig : Inport  Partition=on  PartitionDimension=1  PartitionWidth=1  PartitionOffset=0  BusOutputAsStruct=on
  For Each : ForEach  DisableCoverage=on
  Terminator : Terminator
  wires:
  VehicleConfig/1 -> Terminator/1

== system BEML_EMU_CBTCInterface_Lib/CBTCInterface/CBTCInterfacingUnit/CBTCModel/ATO/ATO Braking Demand ==
  SpeedError : Inport
  Tuning : Inport  Port=2
  Action Port : ActionPort  InitializeStates=reset
  Brake Demand PID Controller : simulink/Continuous/PID Controller  Controller=PID  Form=Parallel  TimeDomain=Discrete-time  SampleTime=-1  IntegratorMethod=Forward Euler  FilterMethod=Forward Euler  ControllerParametersSource=external  P=1  I=1  D=0  UseFilter=off  N=100  TunerSelectOption=Transfer Function Based (PID Tuner App)  InitialConditionSource=internal  InitialConditionForIntegrator=0  InitialConditionForFilter=0  DifferentiatorICPrevScaledInput=0  ExternalReset=none  TrackingMode=off  Kt=1  LimitOutput=on  UpperSaturationLimit=0  LowerSaturationLimit=-100  LinearizeAsGain=off  AntiWindupMode=none  Kb=1  POutMin=[]  POutMax=[]  IOutMin=[]  IOutMax=[]  DOutMin=[]  DOutMax=[]  NOutMin=[]  NOutMax=[]  SumOutMin=[]  SumOutMax=[]  SaturationOutMin=[]  SaturationOutMax=[]  PParamMin=[]  PParamMax=[]  IParamMin=[]  IParamMax=[]  DParamMin=[]  DParamMax=[]  NParamMin=[]  NParamMax=[]  KbParamMin=[]  KbParamMax=[]  KtParamMin=[]  KtParamMax=[]  KbOutMin=[]  KbOutMax=[]  KtOutMin=[]  KtOutMax=[]  IntegratorOutMin=[]  IntegratorOutMax=[]  FilterOutMin=[]  FilterOutMax=[]  SumI1OutMin=[]  SumI1OutMax=[]  SumI2OutMin=[]  SumI2OutMax=[]  SumI3OutMin=[]  SumI3OutMax=[]  SumI4OutMin=[]  SumI4OutMax=[]  SumDOutMin=[]  SumDOutMax=[]  DifferentiatorOutMin=[]  DifferentiatorOutMax=[]  FilterDiffOutCoefMin=[]  FilterDiffOutCoefMax=[]  ReciprocalOutMin=[]  ReciprocalOutMax=[]  SumDenOutMin=[]  SumDenOutMax=[]  SumNumOutMin=[]  SumNumOutMax=[]  DivideOutMin=[]  DivideOutMax=[]  IntegratorContinuousStateAttributes=''  IntegratorStateMustResolveToSignalObject=off  IntegratorRTWStateStorageClass=Auto  FilterContinuousStateAttributes=''  FilterStateMustResolveToSignalObject=off  FilterRTWStateStorageClass=Auto  ParallelPVariant=ExternalParameters  IdealPVariant=Disabled  IVariant=ExternalParameters  DVariant=ExternalParameters  IntegratorVariant=Discrete  SatVariant=Enabled  AWVariant=Passthrough  PCopyVariant=Disabled  TRVariant=Disabled  FdbkBlocksVariant=Forward  IdealPFdbkVariant=Disabled  SatFdbkVariant=Disabled  DerivativeFilterVariant=Differentiator  NVariant=Passthrough  NCopyVariant=Disabled_SignalSpec  FilterICVariant=InternalICsDifferentiator  IntegratorICVariant=InternalICs  ExternalResetVariant=Disabled  TRSumVariant=Passthrough  SumFdbkVariant=Disabled  SumVariant=Sum_PID
  Bus Selector : BusSelector  OutputSignals=ATOBrakeP,ATOBrakeI,ATOBrakeD
  Out1 : Outport  VectorParamsAs1DForOutWhenUnconnected=off
  wires:
  Bus Selector/2 -> Brake Demand PID Controller/3  "<ATOBrakeI>"
  Bus Selector/1 -> Brake Demand PID Controller/2  "<ATOBrakeP>"
  Bus Selector/3 -> Brake Demand PID Controller/4  "<ATOBrakeD>"
  SpeedError/1 -> Brake Demand PID Controller/1
  Brake Demand PID Controller/1 -> Out1/1
  Tuning/1 -> Bus Selector/1

== system BEML_EMU_CBTCInterface_Lib/CBTCInterface/CBTCInterfacingUnit/CBTCModel/ATO/ATO Traction Demand ==
  SpeedError : Inport
  Tuning : Inport  Port=2
  Action Port : ActionPort  InitializeStates=reset
  Bus Selector : BusSelector  OutputSignals=ATOTractionP,ATOTractionI,ATOTractionD
  Tractive Demand : simulink/Continuous/PID Controller  Controller=PID  Form=Parallel  TimeDomain=Discrete-time  SampleTime=-1  IntegratorMethod=Forward Euler  FilterMethod=Forward Euler  ControllerParametersSource=external  P=1  I=1  D=0  UseFilter=off  N=100  TunerSelectOption=Transfer Function Based (PID Tuner App)  InitialConditionSource=internal  InitialConditionForIntegrator=0  InitialConditionForFilter=0  DifferentiatorICPrevScaledInput=0  ExternalReset=none  TrackingMode=off  Kt=1  LimitOutput=on  UpperSaturationLimit=100  LowerSaturationLimit=0  LinearizeAsGain=off  AntiWindupMode=none  Kb=1  POutMin=[]  POutMax=[]  IOutMin=[]  IOutMax=[]  DOutMin=[]  DOutMax=[]  NOutMin=[]  NOutMax=[]  SumOutMin=[]  SumOutMax=[]  SaturationOutMin=[]  SaturationOutMax=[]  PParamMin=[]  PParamMax=[]  IParamMin=[]  IParamMax=[]  DParamMin=[]  DParamMax=[]  NParamMin=[]  NParamMax=[]  KbParamMin=[]  KbParamMax=[]  KtParamMin=[]  KtParamMax=[]  KbOutMin=[]  KbOutMax=[]  KtOutMin=[]  KtOutMax=[]  IntegratorOutMin=[]  IntegratorOutMax=[]  FilterOutMin=[]  FilterOutMax=[]  SumI1OutMin=[]  SumI1OutMax=[]  SumI2OutMin=[]  SumI2OutMax=[]  SumI3OutMin=[]  SumI3OutMax=[]  SumI4OutMin=[]  SumI4OutMax=[]  SumDOutMin=[]  SumDOutMax=[]  DifferentiatorOutMin=[]  DifferentiatorOutMax=[]  FilterDiffOutCoefMin=[]  FilterDiffOutCoefMax=[]  ReciprocalOutMin=[]  ReciprocalOutMax=[]  SumDenOutMin=[]  SumDenOutMax=[]  SumNumOutMin=[]  SumNumOutMax=[]  DivideOutMin=[]  DivideOutMax=[]  IntegratorContinuousStateAttributes=''  IntegratorStateMustResolveToSignalObject=off  IntegratorRTWStateStorageClass=Auto  FilterContinuousStateAttributes=''  FilterStateMustResolveToSignalObject=off  FilterRTWStateStorageClass=Auto  ParallelPVariant=ExternalParameters  IdealPVariant=Disabled  IVariant=ExternalParameters  DVariant=ExternalParameters  IntegratorVariant=Discrete  SatVariant=Enabled  AWVariant=Passthrough  PCopyVariant=Disabled  TRVariant=Disabled  FdbkBlocksVariant=Forward  IdealPFdbkVariant=Disabled  SatFdbkVariant=Disabled  DerivativeFilterVariant=Differentiator  NVariant=Passthrough  NCopyVariant=Disabled_SignalSpec  FilterICVariant=InternalICsDifferentiator  IntegratorICVariant=InternalICs  ExternalResetVariant=Disabled  TRSumVariant=Passthrough  SumFdbkVariant=Disabled  SumVariant=Sum_PID
  Out1 : Outport  VectorParamsAs1DForOutWhenUnconnected=off
  wires:
  SpeedError/1 -> Tractive Demand/1
  Bus Selector/1 -> Tractive Demand/2  "<ATOTractionP>"
  Bus Selector/2 -> Tractive Demand/3  "<ATOTractionI>"
  Tractive Demand/1 -> Out1/1
  Bus Selector/3 -> Tractive Demand/4  "<ATOTractionD>"
  Tuning/1 -> Bus Selector/1

== system BEML_EMU_CBTCInterface_Lib/CBTCInterface/CBTCInterfacingUnit/CBTCModel/ATO/Brake When Close to Stopping Point ==
  Action Port : ActionPort
  Constant : Constant  Value=-100
  Out1 : Outport
  wires:
  Constant/1 -> Out1/1

== system BEML_EMU_CBTCInterface_Lib/CBTCInterface/CBTCInterfacingUnit/CBTCModel/ATO/Coasting ==
  Action Port : ActionPort
  Constant : Constant  Value=0
  Out1 : Outport
  wires:
  Constant/1 -> Out1/1

== system BEML_EMU_CBTCInterface_Lib/CBTCInterface/CBTCInterfacingUnit/CBTCModel/ATO/NotInATO ==
  Action Port : ActionPort
  Constant : Constant  Value=0
  Out1 : Outport
  wires:
  Constant/1 -> Out1/1

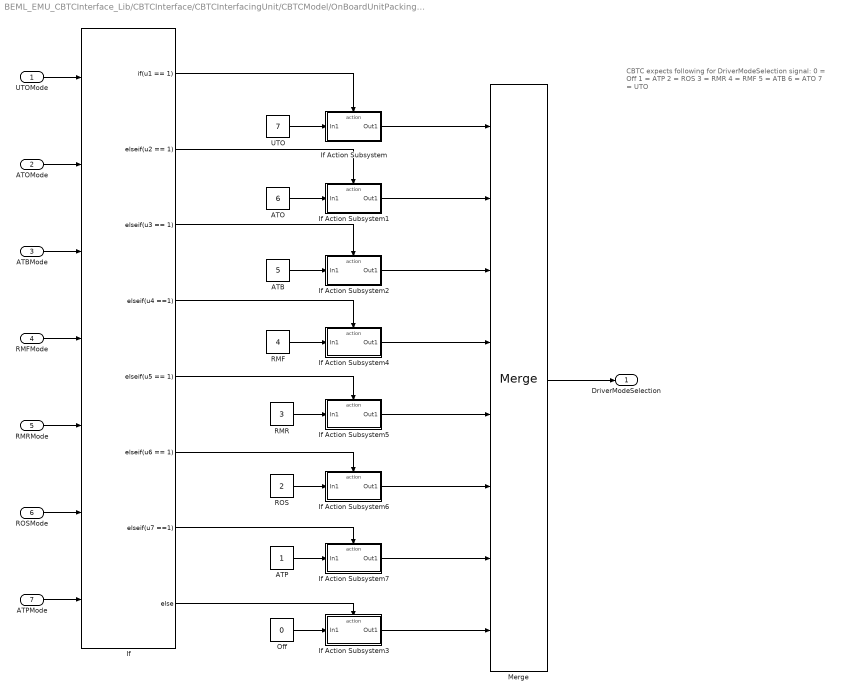
== system BEML_EMU_CBTCInterface_Lib/CBTCInterface/CBTCInterfacingUnit/CBTCModel/OnBoardUnitPacking/DriverModeStatus ==
  note: CBTC expects following for DriverModeSelection signal:
      | 0 = Off
      | 1 = ATP
      | 2 = ROS
      | 3 = RMR
      | 4 = RMF
      | 5 = ATB
      | 6 = ATO
      | 7 = UTO
  UTOMode : Inport
  ATOMode : Inport  Port=2
  ATBMode : Inport  Port=3
  RMFMode : Inport  Port=4
  RMRMode : Inport  Port=5
  ROSMode : Inport  Port=6
  ATPMode : Inport  Port=7
  ATB : Constant  Value=5
  ATO : Constant  Value=6
  ATP : Constant
  If : If  NumInputs=7  IfExpression=u1 == 1  ElseIfExpressions=u2 == 1, u3 == 1, u4 ==1, u5 == 1, u6 == 1, u7 ==1
  If Action Subsystem : Subsystem  TreatAsAtomicUnit=on
  If Action Subsystem1 : Subsystem  TreatAsAtomicUnit=on
  If Action Subsystem2 : Subsystem  TreatAsAtomicUnit=on
  If Action Subsystem3 : Subsystem  TreatAsAtomicUnit=on
  If Action Subsystem4 : Subsystem  TreatAsAtomicUnit=on
  If Action Subsystem5 : Subsystem  TreatAsAtomicUnit=on
  If Action Subsystem6 : Subsystem  TreatAsAtomicUnit=on
  If Action Subsystem7 : Subsystem  TreatAsAtomicUnit=on
  Merge : Merge  Inputs=8
  Off : Constant  Value=0
  RMF : Constant  Value=4
  RMR : Constant  Value=3
  ROS : Constant  Value=2
  UTO : Constant  Value=7
  DriverModeSelection : Outport
  wires:
  RMF/1 -> If Action Subsystem4/1(In1)
  RMR/1 -> If Action Subsystem5/1(In1)
  ROS/1 -> If Action Subsystem6/1(In1)
  ATP/1 -> If Action Subsystem7/1(In1)
  If Action Subsystem7/1(Out1) -> Merge/7
  If Action Subsystem6/1(Out1) -> Merge/6
  If Action Subsystem5/1(Out1) -> Merge/5
  If Action Subsystem4/1(Out1) -> Merge/4
  If/7 -> If Action Subsystem7/Action
  If/6 -> If Action Subsystem6/Action
  If/5 -> If Action Subsystem5/Action
  If/4 -> If Action Subsystem4/Action
  ATPMode/1 -> If/7
  ROSMode/1 -> If/6
  RMRMode/1 -> If/5
  RMFMode/1 -> If/4
  ATBMode/1 -> If/3
  ATOMode/1 -> If/2
  UTOMode/1 -> If/1
  If/1 -> If Action Subsystem/Action
  If/2 -> If Action Subsystem1/Action
  If/3 -> If Action Subsystem2/Action
  If/8 -> If Action Subsystem3/Action
  If Action Subsystem/1(Out1) -> Merge/1
  If Action Subsystem1/1(Out1) -> Merge/2
  If Action Subsystem2/1(Out1) -> Merge/3
  If Action Subsystem3/1(Out1) -> Merge/8
  Merge/1 -> DriverModeSelection/1
  UTO/1 -> If Action Subsystem/1(In1)
  ATO/1 -> If Action Subsystem1/1(In1)
  Off/1 -> If Action Subsystem3/1(In1)
  ATB/1 -> If Action Subsystem2/1(In1)

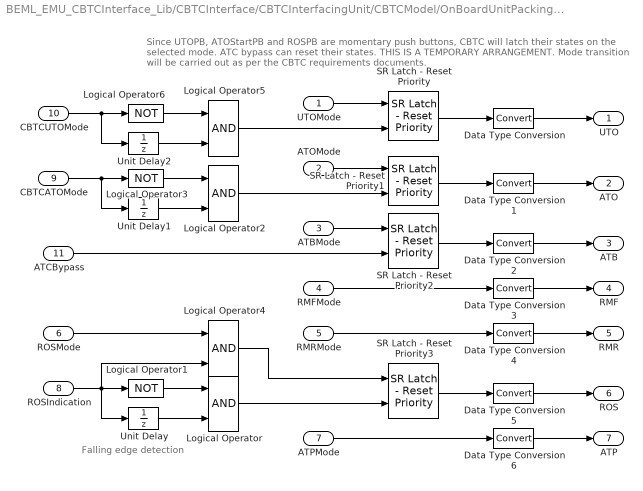
== system BEML_EMU_CBTCInterface_Lib/CBTCInterface/CBTCInterfacingUnit/CBTCModel/OnBoardUnitPacking/ModeLatching ==
  note: Since UTOPB, ATOStartPB and ROSPB are momentary push buttons, CBTC will latch their states on the selected mode.
      | ATC bypass can reset their states.
      | THIS IS A TEMPORARY ARRANGEMENT. Mode transition will be carried out as per the CBTC requirements documents.
  note: Falling edge detection
  UTOMode : Inport
  ATOMode : Inport  Port=2
  ATBMode : Inport  Port=3
  RMFMode : Inport  Port=4
  RMRMode : Inport  Port=5
  ROSMode : Inport  Port=6
  ATPMode : Inport  Port=7
  ROSIndication : Inport  Port=8
  CBTCATOMode : Inport  Port=9
  CBTCUTOMode : Inport  Port=10
  ATCBypass : Inport  Port=11
  Data Type Conversion{,1..6} (7 alike) : DataTypeConversion
  Logical Operator{,2,4..5} (4 alike) : Logic  AllPortsSameDT=off  OutDataTypeStr=boolean
  Logical Operator1 : Logic  Operator=NOT  AllPortsSameDT=off  OutDataTypeStr=boolean
  Logical Operator3 : Logic  Operator=NOT  AllPortsSameDT=off  OutDataTypeStr=boolean
  Logical Operator6 : Logic  Operator=NOT  AllPortsSameDT=off  OutDataTypeStr=boolean
  SR Latch - Reset Priority{,1..3} (4 alike) : LatchesLib/SR Latch - Reset Priority  initial_condition=0
      settings: SourceProductName=Latches
  Unit Delay : UnitDelay  SampleTime=-1  HasFrameUpgradeWarning=on
  Unit Delay1 : UnitDelay  SampleTime=-1  HasFrameUpgradeWarning=on
  Unit Delay2 : UnitDelay  SampleTime=-1  HasFrameUpgradeWarning=on
  UTO : Outport
  ATO : Outport  Port=2
  ATB : Outport  Port=3
  RMF : Outport  Port=4
  RMR : Outport  Port=5
  ROS : Outport  Port=6
  ATP : Outport  Port=7
  wires:
  Logical Operator5/1 -> SR Latch - Reset Priority/2
  Logical Operator6/1 -> Logical Operator5/1
  CBTCUTOMode/1 -> Logical Operator6/1, Unit Delay2/1
  Unit Delay2/1 -> Logical Operator5/2
  Logical Operator4/1 -> SR Latch - Reset Priority3/1
  Unit Delay1/1 -> Logical Operator2/2
  CBTCATOMode/1 -> Unit Delay1/1, Logical Operator3/1
  Logical Operator3/1 -> Logical Operator2/1
  Logical Operator2/1 -> SR Latch - Reset Priority1/2
  Logical Operator/1 -> SR Latch - Reset Priority3/2
  Logical Operator1/1 -> Logical Operator/1
  ROSIndication/1 -> Logical Operator1/1, Unit Delay/1, Logical Operator4/2
  Unit Delay/1 -> Logical Operator/2
  Data Type Conversion6/1 -> ATP/1
  Data Type Conversion5/1 -> ROS/1
  Data Type Conversion4/1 -> RMR/1
  Data Type Conversion3/1 -> RMF/1
  Data Type Conversion2/1 -> ATB/1
  Data Type Conversion1/1 -> ATO/1
  Data Type Conversion/1 -> UTO/1
  ATCBypass/1 -> SR Latch - Reset Priority2/2
  SR Latch - Reset Priority/1 -> Data Type Conversion/1
  SR Latch - Reset Priority1/1 -> Data Type Conversion1/1
  SR Latch - Reset Priority2/1 -> Data Type Conversion2/1
  SR Latch - Reset Priority3/1 -> Data Type Conversion5/1
  UTOMode/1 -> SR Latch - Reset Priority/1
  ATOMode/1 -> SR Latch - Reset Priority1/1
  ATBMode/1 -> SR Latch - Reset Priority2/1
  RMFMode/1 -> Data Type Conversion3/1
  RMRMode/1 -> Data Type Conversion4/1
  ROSMode/1 -> Logical Operator4/1
  ATPMode/1 -> Data Type Conversion6/1

== system BEML_EMU_CBTCInterface_Lib/CBTCInterface/CBTCInterfacingUnit/CBTCModel/OnBoardUnitPacking/DriverModeStatus/If Action Subsystem ==
  In1 : Inport
  Action Port : ActionPort
  Out1 : Outport
  wires:
  In1/1 -> Out1/1

== system BEML_EMU_CBTCInterface_Lib/CBTCInterface/CBTCInterfacingUnit/CBTCModel/OnBoardUnitPacking/DriverModeStatus/If Action Subsystem1 ==
  In1 : Inport
  Action Port : ActionPort
  Out1 : Outport
  wires:
  In1/1 -> Out1/1

== system BEML_EMU_CBTCInterface_Lib/CBTCInterface/CBTCInterfacingUnit/CBTCModel/OnBoardUnitPacking/DriverModeStatus/If Action Subsystem2 ==
  In1 : Inport
  Action Port : ActionPort
  Out1 : Outport
  wires:
  In1/1 -> Out1/1

== system BEML_EMU_CBTCInterface_Lib/CBTCInterface/CBTCInterfacingUnit/CBTCModel/OnBoardUnitPacking/DriverModeStatus/If Action Subsystem3 ==
  In1 : Inport
  Action Port : ActionPort
  Out1 : Outport
  wires:
  In1/1 -> Out1/1

== system BEML_EMU_CBTCInterface_Lib/CBTCInterface/CBTCInterfacingUnit/CBTCModel/OnBoardUnitPacking/DriverModeStatus/If Action Subsystem4 ==
  In1 : Inport
  Action Port : ActionPort
  Out1 : Outport
  wires:
  In1/1 -> Out1/1

== system BEML_EMU_CBTCInterface_Lib/CBTCInterface/CBTCInterfacingUnit/CBTCModel/OnBoardUnitPacking/DriverModeStatus/If Action Subsystem5 ==
  In1 : Inport
  Action Port : ActionPort
  Out1 : Outport
  wires:
  In1/1 -> Out1/1

== system BEML_EMU_CBTCInterface_Lib/CBTCInterface/CBTCInterfacingUnit/CBTCModel/OnBoardUnitPacking/DriverModeStatus/If Action Subsystem6 ==
  In1 : Inport
  Action Port : ActionPort
  Out1 : Outport
  wires:
  In1/1 -> Out1/1

== system BEML_EMU_CBTCInterface_Lib/CBTCInterface/CBTCInterfacingUnit/CBTCModel/OnBoardUnitPacking/DriverModeStatus/If Action Subsystem7 ==
  In1 : Inport
  Action Port : ActionPort
  Out1 : Outport
  wires:
  In1/1 -> Out1/1
